simulink model "CO2"  (R2026a)
settings: Solver=FixedStepDiscrete  FixedStep=0.1
settings Model: Creator=Educação  LastModifiedBy=mateu

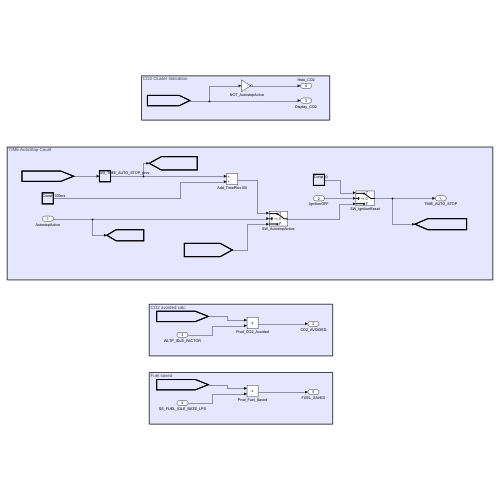
[thumbnail: Simulink's stored preview of the top-level diagram]
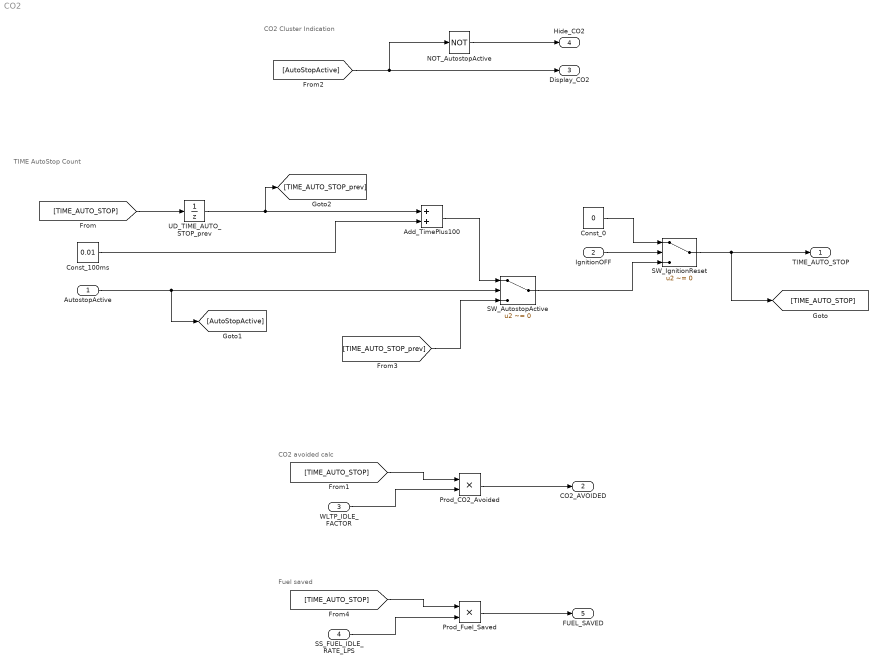
== system CO2 ==
  note: CO2 Cluster Indication
  note: CO2 avoided calc
  note: TIME AutoStop Count
  note: Fuel saved
  AutostopActive : Inport  OutDataTypeStr=boolean
  IgnitionOFF : Inport  Port=2  OutDataTypeStr=boolean
  WLTP_IDLE_FACTOR : Inport  Port=3
  SS_FUEL_IDLE_RATE_LPS : Inport  Port=4
  Add_TimePlus100 : Sum
  Const_0 : Constant  Value=0
  Const_100ms : Constant  Value=0.01
  NOT_AutostopActive : Logic  Operator=NOT  IconShape=distinctive  AllPortsSameDT=off  OutDataTypeStr=boolean
  Prod_CO2_Avoided : Product
  Prod_Fuel_Saved : Product
  SW_AutostopActive : Switch  Criteria=u2 ~= 0  SaturateOnIntegerOverflow=off  InputSameDT=off
  SW_IgnitionReset : Switch  Criteria=u2 ~= 0  SaturateOnIntegerOverflow=off  InputSameDT=off
  UD_TIME_AUTO_STOP_prev : UnitDelay  SampleTime=-1
  TIME_AUTO_STOP : Outport
  CO2_AVOIDED : Outport  Port=2
  Display_CO2 : Outport  Port=3
  Hide_CO2 : Outport  Port=4
  FUEL_SAVED : Outport  Port=5
  wires:
  IgnitionOFF/1 -> SW_IgnitionReset/2
  [TIME_AUTO_STOP_prev] -> SW_AutostopActive/3
  SW_AutostopActive/1 -> SW_IgnitionReset/3
  [TIME_AUTO_STOP] -> Prod_CO2_Avoided/1
  AutostopActive/1 -> SW_AutostopActive/2, [AutoStopActive]
  Prod_CO2_Avoided/1 -> CO2_AVOIDED/1
  Const_100ms/1 -> Add_TimePlus100/2
  UD_TIME_AUTO_STOP_prev/1 -> [TIME_AUTO_STOP_prev], Add_TimePlus100/1
  [TIME_AUTO_STOP] -> UD_TIME_AUTO_STOP_prev/1
  NOT_AutostopActive/1 -> Hide_CO2/1
  WLTP_IDLE_FACTOR/1 -> Prod_CO2_Avoided/2
  [AutoStopActive] -> Display_CO2/1, NOT_AutostopActive/1
  Const_0/1 -> SW_IgnitionReset/1
  Add_TimePlus100/1 -> SW_AutostopActive/1
  SW_IgnitionReset/1 -> [TIME_AUTO_STOP], TIME_AUTO_STOP/1
  Prod_Fuel_Saved/1 -> FUEL_SAVED/1
  [TIME_AUTO_STOP] -> Prod_Fuel_Saved/1
  SS_FUEL_IDLE_RATE_LPS/1 -> Prod_Fuel_Saved/2
